simulink model "test"  (R2024b)
settings: Solver=VariableStepAuto  StartTime=0.0  StopTime=10.0  RelTol=1e-3
libraries: simulink_extras x1
(part 2 of 2)

== system test/buffer22 ==
  In1 : Inport
  Out1 : Outport
  wires:
  In1/1 -> Out1/1

== system test/buffer23 ==
  In1 : Inport
  Out1 : Outport
  wires:
  In1/1 -> Out1/1

== system test/buffer24 ==
  In1 : Inport
  Out1 : Outport
  wires:
  In1/1 -> Out1/1

== system test/buffer25 ==
  In1 : Inport
  Out1 : Outport
  wires:
  In1/1 -> Out1/1

== system test/buffer26 ==
  In1 : Inport
  Out1 : Outport
  wires:
  In1/1 -> Out1/1

== system test/buffer27 ==
  In1 : Inport
  Out1 : Outport
  wires:
  In1/1 -> Out1/1

== system test/buffer28 ==
  In1 : Inport
  Out1 : Outport
  wires:
  In1/1 -> Out1/1

== system test/buffer29 ==
  In1 : Inport
  Out1 : Outport
  wires:
  In1/1 -> Out1/1

== system test/buffer3 ==
  In1 : Inport
  Out1 : Outport
  wires:
  In1/1 -> Out1/1

== system test/buffer30 ==
  In1 : Inport
  Out1 : Outport
  wires:
  In1/1 -> Out1/1

== system test/buffer31 ==
  In1 : Inport
  Out1 : Outport
  wires:
  In1/1 -> Out1/1

== system test/buffer32 ==
  In1 : Inport
  Out1 : Outport
  wires:
  In1/1 -> Out1/1

== system test/buffer33 ==
  In1 : Inport
  Out1 : Outport
  wires:
  In1/1 -> Out1/1

== system test/buffer34 ==
  In1 : Inport
  Out1 : Outport
  wires:
  In1/1 -> Out1/1

== system test/buffer35 ==
  In1 : Inport
  Out1 : Outport
  wires:
  In1/1 -> Out1/1

== system test/buffer36 ==
  In1 : Inport
  Out1 : Outport
  wires:
  In1/1 -> Out1/1

== system test/buffer37 ==
  In1 : Inport
  Out1 : Outport
  wires:
  In1/1 -> Out1/1

== system test/buffer38 ==
  In1 : Inport
  Out1 : Outport
  wires:
  In1/1 -> Out1/1

== system test/buffer39 ==
  In1 : Inport
  Out1 : Outport
  wires:
  In1/1 -> Out1/1

== system test/buffer4 ==
  In1 : Inport
  Out1 : Outport
  wires:
  In1/1 -> Out1/1

== system test/buffer40 ==
  In1 : Inport
  Out1 : Outport
  wires:
  In1/1 -> Out1/1

== system test/buffer41 ==
  In1 : Inport
  Out1 : Outport
  wires:
  In1/1 -> Out1/1

== system test/buffer42 ==
  In1 : Inport
  Out1 : Outport
  wires:
  In1/1 -> Out1/1

== system test/buffer43 ==
  In1 : Inport
  Out1 : Outport
  wires:
  In1/1 -> Out1/1

== system test/buffer44 ==
  In1 : Inport
  Out1 : Outport
  wires:
  In1/1 -> Out1/1

== system test/buffer45 ==
  In1 : Inport
  Out1 : Outport
  wires:
  In1/1 -> Out1/1

== system test/buffer5 ==
  In1 : Inport
  Out1 : Outport
  wires:
  In1/1 -> Out1/1

== system test/buffer6 ==
  In1 : Inport
  Out1 : Outport
  wires:
  In1/1 -> Out1/1

== system test/buffer7 ==
  In1 : Inport
  Out1 : Outport
  wires:
  In1/1 -> Out1/1

== system test/buffer8 ==
  In1 : Inport
  Out1 : Outport
  wires:
  In1/1 -> Out1/1

== system test/buffer9 ==
  In1 : Inport
  Out1 : Outport
  wires:
  In1/1 -> Out1/1
